simulink model "Sim3"  (R2022a)
settings: Solver=VariableStepAuto  StartTime=0.0  StopTime=100  RelTol=1e-3
undefined symbols (not defined in the file): Af, Am, Bf, Bm, Cf, Cm, Df, Dm
settings Model: Creator=Joseph  LastModifiedBy=Joseph

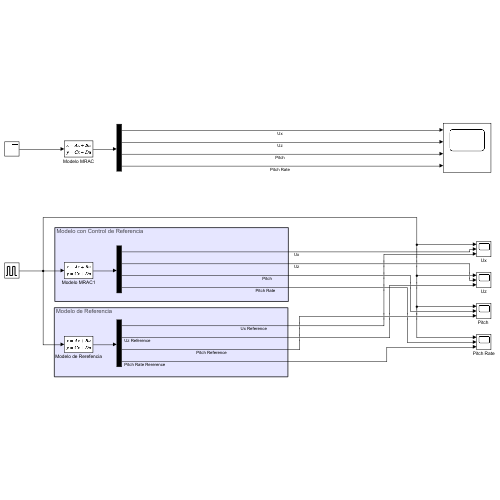
[thumbnail: Simulink's stored preview of the top-level diagram]
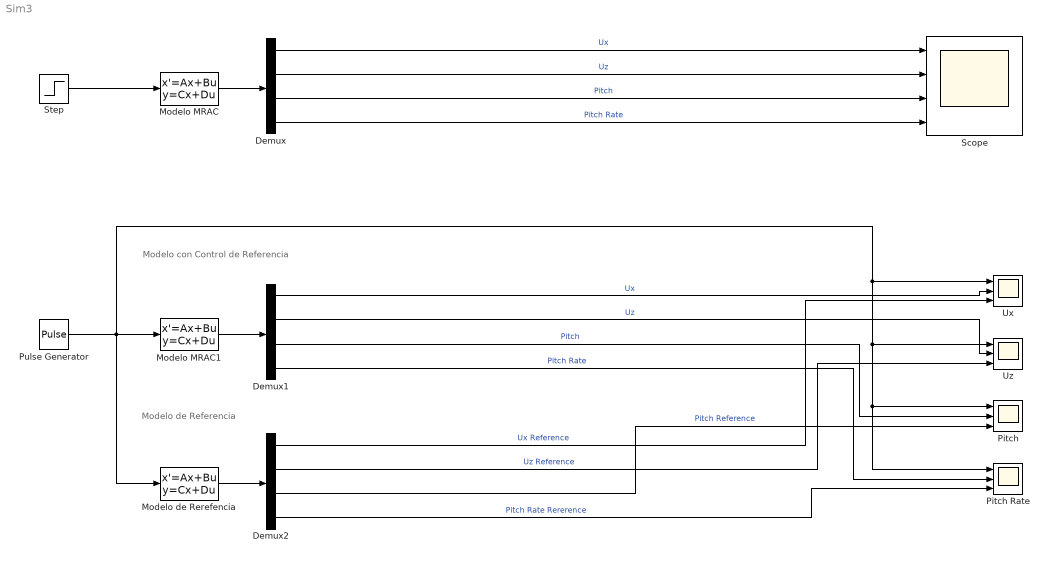
== system Sim3 ==
  note: Modelo de Referencia
  note: Modelo con Control de Referencia
  Demux : Demux
  Demux1 : Demux
  Demux2 : Demux
  Modelo MRAC : StateSpace  A=Af  B=Bf  C=Cf  D=Df  InitialCondition=0
  Modelo MRAC1 : StateSpace  A=Af  B=Bf  C=Cf  D=Df  InitialCondition=0
  Modelo de Rerefencia : StateSpace  A=Am  B=Bm  C=Cm  D=Dm  InitialCondition=0
  "Pitch " : Scope  NumInputPorts=3
  Pitch Rate : Scope  NumInputPorts=3
  Pulse Generator : DiscretePulseGenerator  PulseType=Time based  Period=10  PulseWidth=50  PhaseDelay=5
  Scope : Scope  NumInputPorts=4
  Step : Step  Time=0  SampleTime=0  ZeroCross=off
  Ux : Scope  NumInputPorts=3
  Uz : Scope  NumInputPorts=3
  wires:
  Step/1 -> Modelo MRAC/1
  Modelo MRAC/1 -> Demux/1
  Demux/1 -> Scope/1  "Ux"
  Demux/3 -> Scope/3  "Pitch"
  Demux/2 -> Scope/2  "Uz"
  Demux/4 -> Scope/4  "Pitch Rate"
  Demux1/1 -> Ux/2  "Ux"
  Demux1/2 -> Uz/2  "Uz"
  Demux1/4 -> Pitch Rate/2  "Pitch Rate"
  Demux1/3 -> "Pitch "/2  "Pitch"
  Modelo MRAC1/1 -> Demux1/1
  Pulse Generator/1 -> Modelo de Rerefencia/1, Ux/1, Uz/1, Pitch Rate/1, "Pitch "/1, Modelo MRAC1/1
  Modelo de Rerefencia/1 -> Demux2/1
  Demux2/3 -> "Pitch "/3  "Pitch Reference"
  Demux2/4 -> Pitch Rate/3  "Pitch Rate Rererence"
  Demux2/1 -> Ux/3  "Ux Reference"
  Demux2/2 -> Uz/3  "Uz Reference"
